simulink model "het_platoon_model"  (R2018b)
settings: Solver=ode1  StartTime=0.0  StopTime=simDrv.time_s(end)  FixedStep=sim_t_step  RelTol=1e-3
values from neighbouring files (symbols this model uses):
  sim_t_step = 0.01    [startHetPlatoonModel.m]
undefined symbols (not defined in the file or in its folder): adj_motEffMap, CTModel, DiscIntNeverNeededParam, LT, motSpdVec, motTrqVec, msk_mot_cont_trq, msk_mot_num, msk_mot_spd_bpt, MT, N_OptResults, simDrv, SPHETModel, TT
libraries: platooning_custom_blocks x24, simulink x7, dspstat3 x1, custom_func x1
(part 2 of 3)

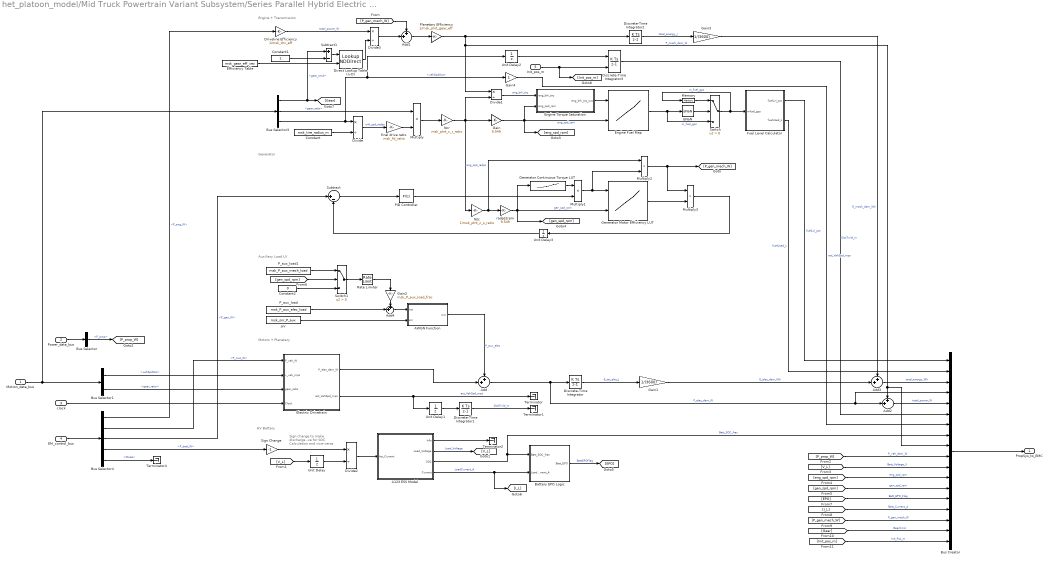
== system het_platoon_model/Mid Truck Powertrain Variant Subsystem/Series Parallel Hybrid Electric Truck/Series Parallel Hybrid Electric Powertrain Power Loss Model ==
  note: Sign change to make discharge -ve
      | for SOC Calculation and vice-versa
  note: Engine + Transmission
  note: HV Battery
  note: Auxiliary Load LV
  note: Motors + Planetary
  note: Generator
  Motion_data_bus : Inport
  Power_data_bus : Inport  Port=2
  clock : Inport  Port=3
  EM_control_bus : Inport  Port=4
  Init_pos_m : Inport  Port=5
  A123 ESS Model : Subsystem
  AWGN Function : MATLAB Function  TreatAsAtomicUnit=on
  Add{,1..4} (5 alike) : Sum  Inputs=++|
  Battery EPO Logic : Subsystem
  Bus Creator : BusCreator  Inputs=18
  Bus Selector : BusSelector  OutputSignals=P_prop
  Bus Selector1 : BusSelector  OutputSignals=vehSpdOut,gear_ratio
  Bus Selector3 : BusSelector  OutputSignals=gear_cmd,gear_ratio,vehSpdOut
  Bus Selector4 : BusSelector  OutputSignals=P_eng_W,P_mot_W,P_gen_W,P_batt_W,Mode
  Constant : Constant  Value=msk_tire_radius_m
  Constant1 : Constant
  Constant2 : Constant  Value=0
  Direct Lookup Table (n-D) : LookupNDDirect  NumberOfTableDimensions=1  TableIsInput=on
  Discrete-Time Integrator : DiscreteIntegrator  SampleTime=msk_t_step  ICPrevOutput=DiscIntNeverNeededParam  ICPrevScaledInput=DiscIntNeverNeededParam
  Discrete-Time Integrator1 : DiscreteIntegrator  SampleTime=msk_t_step  ICPrevOutput=DiscIntNeverNeededParam  ICPrevScaledInput=DiscIntNeverNeededParam
  Discrete-Time Integrator2 : DiscreteIntegrator  SampleTime=-1  ICPrevOutput=DiscIntNeverNeededParam  ICPrevScaledInput=DiscIntNeverNeededParam
  Discrete-Time Integrator3 : DiscreteIntegrator  InitialConditionSource=external  SampleTime=msk_t_step  ICPrevOutput=DiscIntNeverNeededParam  ICPrevScaledInput=DiscIntNeverNeededParam
  Divide{,1..3} (4 alike) : Product  Inputs=*/
  Driveline Efficiency : Gain  Gain=1/msk_drv_eff
  Efficiency Table : Constant  Value=msk_gear_eff_vec
  Electric Drivetrain : Subsystem
  Engine Fuel Map : Lookup_n-D  BreakpointsForDimension1=msk_eng_trq_bpt  BreakpointsForDimension2=msk_eng_spd_bpt  Table=msk_eng_fuel_map  ExtrapMethod=Clip  UseLastTableValue=on  InternalRulePriority=Speed  RndMeth=Simplest  InputSameDT=on
  Engine Torque Saturation : Subsystem
  Fuel Level Calculator : Subsystem
  Gain : Gain  Gain=9.549
  Gain1 : Gain  Gain=1/(3600)
  Gain2 : Gain  Gain=msk_P_aux_load_frac
  Gain3 : Gain  Gain=1/(3600)
  Gain4 : Gain
  Generator Continuous Torque LUT : Lookup_n-D  NumberOfTableDimensions=1  BreakpointsForDimension1=msk_gen_mtr_spdbpt  Table=msk_gen_mtr_cont_trq  InternalRulePriority=Speed  RndMeth=Simplest  InputSameDT=on
  Generator Motor Efficiency LUT : Lookup_n-D  BreakpointsForDimension1=msk_gen_mtr_trqbpt  BreakpointsForDimension2=msk_gen_mtr_spdbpt  Table=msk_gen_mtr_eff_map  ExtrapMethod=Clip  UseLastTableValue=on  InternalRulePriority=Speed  RndMeth=Simplest  InputSameDT=on
  IsNaN : RelationalOperator  Operator=isNaN  OutDataTypeStr=boolean  RndMeth=Simplest
  Memory : Memory
  Multiply{,1..3} (4 alike) : Product
  Ncr : Gain  Gain=msk_plnt_c_r_ratio
  Nsc : Gain  Gain=1/msk_plnt_c_s_ratio
  PID Controller : simulink/Continuous/PID Controller  Controller=PI  Form=Parallel  TimeDomain=Discrete-time  SampleTime=-1  IntegratorMethod=Forward Euler  FilterMethod=Forward Euler  ControllerParametersSource=internal  P=msk_gen_ctl_Kp  I=msk_gen_ctl_Ki  D=0  UseFilter=on  N=100  TunerSelectOption=Transfer Function Based (PID Tuner App)  InitialConditionSource=internal  InitialConditionForIntegrator=0  InitialConditionForFilter=0  DifferentiatorICPrevScaledInput=0  ExternalReset=none  TrackingMode=off  Kt=1  LimitOutput=on  UpperSaturationLimit=1  LowerSaturationLimit=0  LinearizeAsGain=on  AntiWindupMode=clamping  Kb=1  POutMin=[]  POutMax=[]  IOutMin=[]  IOutMax=[]  DOutMin=[]  DOutMax=[]  NOutMin=[]  NOutMax=[]  SumOutMin=[]  SumOutMax=[]  SaturationOutMin=[]  SaturationOutMax=[]  PParamMin=[]  PParamMax=[]  IParamMin=[]  IParamMax=[]  DParamMin=[]  DParamMax=[]  NParamMin=[]  NParamMax=[]  KbParamMin=[]  KbParamMax=[]  KtParamMin=[]  KtParamMax=[]  KbOutMin=[]  KbOutMax=[]  KtOutMin=[]  KtOutMax=[]  IntegratorOutMin=[]  IntegratorOutMax=[]  FilterOutMin=[]  FilterOutMax=[]  SumI1OutMin=[]  SumI1OutMax=[]  SumI2OutMin=[]  SumI2OutMax=[]  SumI3OutMin=[]  SumI3OutMax=[]  SumI4OutMin=[]  SumI4OutMax=[]  SumDOutMin=[]  SumDOutMax=[]  DifferentiatorOutMin=[]  DifferentiatorOutMax=[]  FilterDiffOutCoefMin=[]  FilterDiffOutCoefMax=[]  ReciprocalOutMin=[]  ReciprocalOutMax=[]  SumDenOutMin=[]  SumDenOutMax=[]  SumNumOutMin=[]  SumNumOutMax=[]  DivideOutMin=[]  DivideOutMax=[]  IntegratorContinuousStateAttributes=''  IntegratorStateMustResolveToSignalObject=off  IntegratorRTWStateStorageClass=Auto  FilterContinuousStateAttributes=''  FilterStateMustResolveToSignalObject=off  FilterRTWStateStorageClass=Auto  ParallelPVariant=InternalParameters  IdealPVariant=Disabled  IVariant=InternalParameters  DVariant=Disabled  IntegratorVariant=Discrete  SatVariant=Enabled  AWVariant=DiscClampingParallel  PCopyVariant=Disabled  TRVariant=Disabled  FdbkBlocksVariant=Forward  IdealPFdbkVariant=Disabled  SatFdbkVariant=Disabled  DerivativeFilterVariant=Disabled  NVariant=Disabled  NCopyVariant=Disabled_SignalSpec  FilterICVariant=Disabled  IntegratorICVariant=InternalICs  ExternalResetVariant=Disabled  TRSumVariant=Passthrough  SumFdbkVariant=Disabled  SumVariant=Sum_PI
  P_aux_load : Constant  Value=msk_P_aux_elec_load
  P_aux_load1 : Constant  Value=msk_P_aux_mech_load
  Planetary Efficiency : Gain  Gain=1/msk_plnt_gear_eff
  Rate Limiter : RateLimiter  RisingSlewLimit=100  FallingSlewLimit=-100  SampleTimeMode=inherited
  Sign Change : Gain  Gain=-1
  Subtract : Sum  Inputs=|+-
  Subtract1 : Sum  Inputs=+-
  Switch : Switch  Criteria=u2 > Threshold
  Switch1 : Switch  Criteria=u2 > Threshold
  Terminator{,1..2,4} (4 alike) : Terminator
  Unit Delay : UnitDelay  InitialCondition=msk_batt_Ns* msk_batt_Nmod * msk_cell_Vnom  SampleTime=-1
  Unit Delay1 : UnitDelay  SampleTime=-1
  Unit Delay2 : UnitDelay  SampleTime=-1
  Unit Delay3 : UnitDelay  SampleTime=-1
  final drive ratio : Gain  Gain=msk_fd_ratio
  radps2rpm : Gain  Gain=9.549
  snr : Constant  Value=msk_snr_P_aux
  PropSys_to_EMC : Outport
  wires:
  Divide3/1 -> Add1/2
  Bus Selector3/2 -> Multiply/1  "<gear_ratio>"
  Direct Lookup Table (n-D)/1 -> Divide3/2
  Efficiency Table/1 -> Direct Lookup Table (n-D)/2
  Constant1/1 -> Subtract1/2
  Subtract1/1 -> Direct Lookup Table (n-D)/1
  Add3/1 -> Bus Creator/3  "total_energy_Wh"
  Add2/1 -> Bus Creator/5  "total_power_W"
  Add1/1 -> Planetary Efficiency/1
  Bus Selector1/2 -> Electric Drivetrain/3(gear_ratio)  "<gear_ratio>"
  Driveline Efficiency/1 -> Divide3/1  "total_power_W"
  [P_gen_mech_W] -> Add1/1
  Unit Delay3/1 -> Subtract/2
  Multiply3/1 -> Unit Delay3/1
  Multiply2/1 -> Multiply3/1, [P_gen_mech_W]
  Generator Motor Efficiency LUT/1 -> Multiply3/2
  Generator Continuous Torque LUT/1 -> Multiply1/1
  Multiply1/1 -> Generator Motor Efficiency LUT/1, Multiply2/2
  PID Controller/1 -> Multiply1/2
  Subtract/1 -> PID Controller/1
  radps2rpm/1 -> [gen_spd_rpm], Generator Motor Efficiency LUT/2, Generator Continuous Torque LUT/1  "gen_spd_rpm"
  Nsc/1 -> radps2rpm/1, Multiply2/1
  Bus Selector4/2 -> Electric Drivetrain/1(P_veh_W)  "<P_mot_W>"
  Bus Selector/1 -> [P_prop_W]  "<P_prop>"
  EM_control_bus/1 -> Bus Selector4/1
  final drive ratio/1 -> Multiply/2
  Unit Delay2/1 -> Discrete-Time Integrator3/1
  Bus Selector3/3 -> Divide/1, Unit Delay2/1, Gain4/1  "<vehSpdOut>"
  Divide/1 -> final drive ratio/1  "whl_spd_radps"
  Gain4/1 -> Bus Creator/7  "act_VehSpd_mps"
  Discrete-Time Integrator3/1 -> Bus Creator/6  "DistTrvld_m"
  Divide1/1 -> Engine Torque Saturation/1(eng_brk_trq)  "eng_brk_trq"
  Fuel Level Calculator/2(fuelUsed_L) -> Bus Creator/2  "fuelUsed_L"
  Multiply/1 -> Ncr/1
  Discrete-Time Integrator2/1 -> Gain3/1  "total_energy_J"
  Engine Torque Saturation/1(eng_brk_trq_out) -> Engine Fuel Map/1
  Fuel Level Calculator/1(fuelLvl_pct) -> Bus Creator/1  "fuelLvl_pct"
  Motion_data_bus/1 -> Bus Selector1/1, Bus Selector3/1
  Gain3/1 -> Add3/1  "E_mech_dem_Wh"
  Constant/1 -> Divide/2
  Gain/1 -> [eng_spd_rpm], Engine Fuel Map/2, Engine Torque Saturation/2(eng_spd_rpm)  "eng_spd_rpm"
  Unit Delay1/1 -> Discrete-Time Integrator1/1
  Discrete-Time Integrator1/1 -> Terminator1/1  "DistTrvld_m"
  Electric Drivetrain/2(act_VehSpd_mps) -> Unit Delay1/1, Terminator/1  "act_VehSpd_mps"
  A123 ESS Model/4(Current) -> [I_L], Battery EPO Logic/2(LoadCurrent_A)  "LoadCurrent_A"
  Bus Selector4/4 -> Sign Change/1  "<P_batt_W>"
  Sign Change/1 -> Divide2/1
  Battery EPO Logic/1(Batt_EPO) -> [EPO]  "BattEPOFlag"
  Unit Delay/1 -> Divide2/2
  [V_L] -> Unit Delay/1
  A123 ESS Model/1(Info) -> Terminator2/1
  A123 ESS Model/3(SOC) -> Battery EPO Logic/1(Batt_SOC_frac), Bus Creator/8  "Batt_SOC_frac"
  Divide2/1 -> A123 ESS Model/1(Inp_Current)
  A123 ESS Model/2(Load_Voltage) -> [V_L]  "Load_Voltage"
  Gain1/1 -> Add3/2  "E_elec_dem_Wh"
  Discrete-Time Integrator/1 -> Gain1/1  "E_tot_elec_J"
  Bus Creator/1 -> PropSys_to_EMC/1
  Electric Drivetrain/1(P_elec_dem_W) -> Add/2
  Add/1 -> Bus Creator/4, Add2/2, Discrete-Time Integrator/1  "P_elec_dem_W"
  AWGN Function/1(out) -> Add/1  "P_aux_elec"
  snr/1 -> AWGN Function/2(snr)
  P_aux_load/1 -> Add4/2
  Bus Selector1/1 -> Electric Drivetrain/2(v_veh_mps)  "<vehSpdOut>"
  clock/1 -> Electric Drivetrain/4(Clock)
  Power_data_bus/1 -> Bus Selector/1
  Bus Selector3/1 -> Subtract1/1, [Gear]  "<gear_cmd>"
  Switch/1 -> Fuel Level Calculator/1(mfuel_gps), Memory/1  "m_fuel_gps"
  Memory/1 -> Switch/1
  Engine Fuel Map/1 -> Switch/3, IsNaN/1  "m_fuel_gps"
  IsNaN/1 -> Switch/2
  [P_prop_W] -> Bus Creator/10  "P_veh_dem_W"
  Bus Selector4/1 -> Driveline Efficiency/1  "<P_eng_W>"
  Bus Selector4/3 -> Subtract/1  "<P_gen_W>"
  Bus Selector4/5 -> Terminator4/1  "<Mode>"
  [V_L] -> Bus Creator/11  "Batt_Voltage_V"
  Ncr/1 -> Divide1/2, Gain/1, Nsc/1  "eng_spd_radps"
  [gen_spd_rpm] -> Bus Creator/13  "gen_spd_rpm"
  [eng_spd_rpm] -> Bus Creator/12  "eng_spd_rpm"
  Init_pos_m/1 -> [Init_pos_m], Discrete-Time Integrator3/2
  Add4/1 -> AWGN Function/1(inp)
  Gain2/1 -> Add4/1
  P_aux_load1/1 -> Switch1/1
  Switch1/1 -> Rate Limiter/1
  Rate Limiter/1 -> Gain2/1
  [gen_spd_rpm] -> Switch1/2
  Constant2/1 -> Switch1/3
  [Gear] -> Bus Creator/17  "GearCmd"
  [EPO] -> Bus Creator/14  "Batt_EPO_Flag"
  [I_L] -> Bus Creator/15  "Batt_Current_A"
  [P_gen_mech_W] -> Bus Creator/16  "P_gen_mech_W"
  Planetary Efficiency/1 -> Divide1/1, Bus Creator/9, Add2/1, Discrete-Time Integrator2/1  "P_mech_dem_W"
  [Init_pos_m] -> Bus Creator/18  "Init_Pos_m"

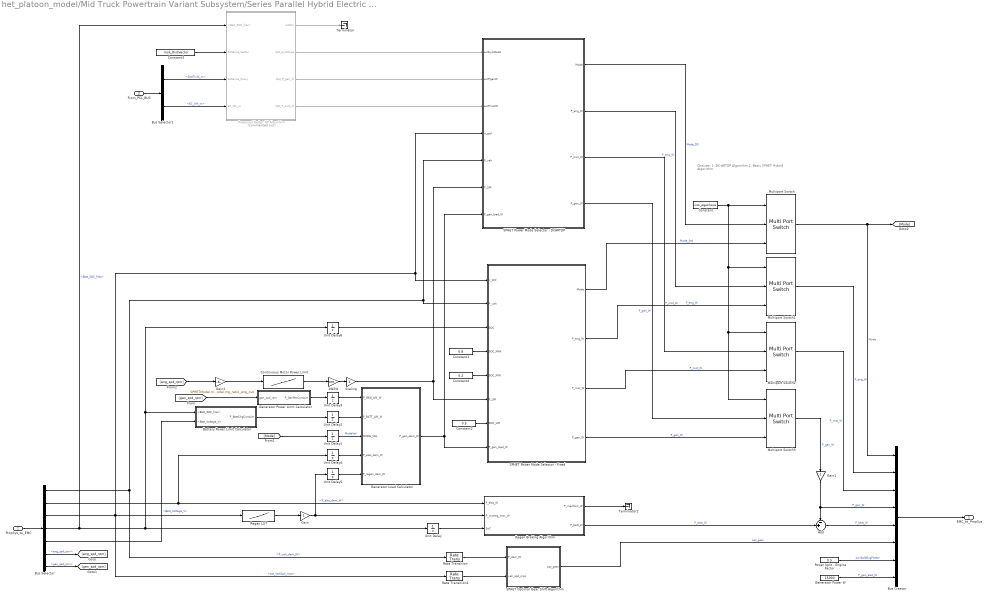
== system het_platoon_model/Mid Truck Powertrain Variant Subsystem/Series Parallel Hybrid Electric Truck/Series Parallel Hybrid Electric Truck Energy Management System ==
  note: Choices:
      | 1: DC-ARTDP Algorithm
      | 2: Basic SPHET Hybrid Algorithm
  PropSys_to_EMC : Inport
  From_PCL_BUS : Inport  Port=2
  Add : Sum  Inputs=-+|
  Battery Power Limit Calculator : Subsystem
  Bus Creator : BusCreator  Inputs=8
  Bus Selector : BusSelector  OutputSignals=P_veh_dem_W,P_elec_dem_W,act_VehSpd_mps,Batt_SOC_frac,Batt_Voltage_V,eng_spd_rpm,gen_spd_rpm
  Bus Selector1 : BusSelector  OutputSignals=DistTrvld_m,EC_Wh_m
  Constant : Constant  Value=msk_algoChoice
  Constant1 : Constant  Value=0.8
  Constant2 : Constant  Value=0.5
  Constant3 : Constant  Value=msk_DistVector
  Constant4 : Constant  Value=0.2
  Continuous Motor Power Limit : Lookup_n-D  NumberOfTableDimensions=1  BreakpointsForDimension1=SPHETModel.cont_mtr_trq_spdbpt  Table=SPHETModel.cont_mtr_pwr_map  InternalRulePriority=Speed  RndMeth=Simplest  InputSameDT=on
  Gain : Gain  Gain=-1
  Gain1 : Gain
  Gain2 : Gain  Gain=SPHETModel.mg_ratio_mot_out/SPHETModel.mg_ratio_eng_out
  Generator Load Calculator : MATLAB Function  TreatAsAtomicUnit=on
  Generator Power Limit Calculator : Subsystem
  Generator Power W : Constant  Value=15000
  Multiport Switch{,1..3} (4 alike) : MultiPortSwitch  Inputs=2
  Power Split - Engine Factor : Constant  Value=0.5
  Proposed ReOpt DP Algorithm : Subsystem  Commented=on
  Rate Transition : RateTransition  OutPortSampleTime=sim_t_step
  Rate Transition1 : RateTransition  OutPortSampleTime=sim_t_step
  Regen Braking Algorithm : Stateflow chart  TreatAsAtomicUnit=on
  Regen LUT : Lookup_n-D  NumberOfTableDimensions=1  BreakpointsForDimension1=msk_regen_spd_bpt  Table=msk_regen_pwr_vec*-1  ExtrapMethod=Clip  UseLastTableValue=on  InternalRulePriority=Speed  RndMeth=Simplest  InputSameDT=on
  SPHET Optimal Gear Shift Algorithm : Subsystem  mask{msk_tire_radius_m=SPHETModel.ld_tire_rad_m, msk_trns_eff_avg=mean(SPHETModel.gear_eff) * SPHETModel.plnt_gear_eff, msk_init_gear=1}
      mask prompts: msk_tire_radius_m "Vehicle tire radius :"; msk_trns_eff_avg "Average transmission efficiency :"; msk_init_gear "Initial gear selection :"
      mask DialogControl DescGroupVar Prompt: Optimal Gear Shift Algorithm
      mask DialogControl DescTextVar Prompt: The block computes optimal gear based on the power demand and vehicle speed by minimizing fuel consumption.
  SPHET Power Mode Selector - DCARTDP : Stateflow chart  TreatAsAtomicUnit=on
  SPHET Power Mode Selector - Fixed : Stateflow chart  TreatAsAtomicUnit=on
  Scaling : Gain
  Terminator : Terminator
  Terminator2 : Terminator
  Unit Delay{,1..6} (7 alike) : UnitDelay  SampleTime=-1
  kW2W : Gain  Gain=1000
  EMC_to_PropSys : Outport
  wires:
  Bus Selector/1 -> SPHET Power Mode Selector - DCARTDP/5(P_veh), SPHET Power Mode Selector - Fixed/2(P_veh), Rate Transition/1  "<P_veh_dem_W>"
  Generator Power W/1 -> Bus Creator/8  "P_gen_elec_W"
  Power Split - Engine Factor/1 -> Bus Creator/7  "pwrSplitEngFactor"
  Bus Creator/1 -> EMC_to_PropSys/1
  From_PCL_BUS/1 -> Bus Selector1/1
  PropSys_to_EMC/1 -> Bus Selector/1
  Bus Selector/4 -> Proposed ReOpt DP Algorithm/1(<Batt_SOC_frac>), Battery Power Limit Calculator/1(<Batt_SOC_frac>), Unit Delay6/1, Unit Delay/1  "<Batt_SOC_frac>"
  Bus Selector/2 -> Regen Braking Algorithm/1(P_elec_W), Unit Delay4/1  "<P_elec_dem_W>"
  Add/1 -> Bus Creator/5  "P_batt_W"
  Regen LUT/1 -> Gain/1
  Regen Braking Algorithm/1(P_mechbrk_W) -> Terminator2/1
  Unit Delay/1 -> Regen Braking Algorithm/3(SoC)
  Bus Selector/3 -> Regen LUT/1, SPHET Power Mode Selector - DCARTDP/4(v_spd), SPHET Power Mode Selector - Fixed/1(v_spd), Rate Transition1/1  "<act_VehSpd_mps>"
  Rate Transition/1 -> SPHET Optimal Gear Shift Algorithm/1(P_dem_W)
  Rate Transition1/1 -> SPHET Optimal Gear Shift Algorithm/2(veh_spd_mps)
  SPHET Optimal Gear Shift Algorithm/1(opt_gear) -> Bus Creator/6  "opt_gear"
  kW2W/1 -> Scaling/1
  Constant1/1 -> SPHET Power Mode Selector - Fixed/4(SOC_MAX)
  Constant2/1 -> SPHET Power Mode Selector - Fixed/7(SOC_LIM)
  Multiport Switch/1 -> Bus Creator/1, [Mode]  "Mode"
  Regen Braking Algorithm/2(P_batt_W) -> Add/2  "P_batt_W"
  Multiport Switch3/1 -> Gain1/1  "P_gen_W"
  Multiport Switch1/1 -> Bus Creator/2  "P_eng_W"
  Multiport Switch2/1 -> Bus Creator/3  "P_mot_W"
  Generator Load Calculator/1(P_gen_dem_W) -> SPHET Power Mode Selector - DCARTDP/7(P_gen_load_W), SPHET Power Mode Selector - Fixed/8(P_gen_load_W)
  Bus Selector/6 -> [eng_spd_rpm]  "<eng_spd_rpm>"
  Bus Selector/7 -> [gen_spd_rpm]  "<gen_spd_rpm>"
  [Mode] -> Unit Delay1/1
  Unit Delay1/1 -> Generator Load Calculator/3(MODE_VAL)  "ModeVal"
  Bus Selector/5 -> Battery Power Limit Calculator/2(<Batt_Voltage_V>)  "<Batt_Voltage_V>"
  Battery Power Limit Calculator/1(P_BattChgContLim) -> Unit Delay2/1
  [gen_spd_rpm] -> Generator Power Limit Calculator/1(gen_spd_rpm)
  Generator Power Limit Calculator/1(P_GenMtrContLim) -> Unit Delay3/1
  Gain/1 -> Regen Braking Algorithm/2(P_motreg_max_W), Unit Delay5/1
  Gain1/1 -> Add/1, Bus Creator/4  "P_gen_W"
  Unit Delay2/1 -> Generator Load Calculator/2(P_BATT_LIM_W)
  Unit Delay3/1 -> Generator Load Calculator/1(P_GEN_LIM_W)
  Unit Delay4/1 -> Generator Load Calculator/4(P_elec_dem_W)
  Unit Delay5/1 -> Generator Load Calculator/5(P_regen_dem_W)
  Unit Delay6/1 -> SPHET Power Mode Selector - Fixed/3(SOC)
  Continuous Motor Power Limit/1 -> kW2W/1
  Gain2/1 -> Continuous Motor Power Limit/1
  [eng_spd_rpm] -> Gain2/1
  SPHET Power Mode Selector - Fixed/4(P_gen_W) -> Multiport Switch3/3  "P_gen_W"
  SPHET Power Mode Selector - Fixed/3(P_mot_W) -> Multiport Switch2/3  "P_mot_W"
  SPHET Power Mode Selector - Fixed/2(P_eng_W) -> Multiport Switch1/3  "P_eng_W"
  SPHET Power Mode Selector - Fixed/1(Mode) -> Multiport Switch/3  "Mode_Std"
  SPHET Power Mode Selector - DCARTDP/4(P_gen_W) -> Multiport Switch3/2  "P_gen_W"
  SPHET Power Mode Selector - DCARTDP/3(P_mot_W) -> Multiport Switch2/2  "P_mot_W"
  SPHET Power Mode Selector - DCARTDP/2(P_eng_W) -> Multiport Switch1/2  "P_eng_W"
  SPHET Power Mode Selector - DCARTDP/1(Mode) -> Multiport Switch/2  "Mode_DC"
  Constant/1 -> Multiport Switch3/1, Multiport Switch2/1, Multiport Switch1/1, Multiport Switch/1
  Bus Selector1/2 -> Proposed ReOpt DP Algorithm/4(EC_Wh_m)  "<EC_Wh_m>"
  Bus Selector1/1 -> Proposed ReOpt DP Algorithm/3(Distance_Query)  "<DistTrvld_m>"
  Proposed ReOpt DP Algorithm/4(Opt_P_mot_W) -> SPHET Power Mode Selector - DCARTDP/3(extPmotW)
  Proposed ReOpt DP Algorithm/2(Opt_HybMode) -> SPHET Power Mode Selector - DCARTDP/1(extHybMode)
  Proposed ReOpt DP Algorithm/3(Opt_P_gen_W) -> SPHET Power Mode Selector - DCARTDP/2(extPgenW)
  Proposed ReOpt DP Algorithm/1(distIdx) -> Terminator/1
  Constant3/1 -> Proposed ReOpt DP Algorithm/2(Distance_Vector)
  Scaling/1 -> SPHET Power Mode Selector - DCARTDP/6(P_LIM), SPHET Power Mode Selector - Fixed/6(P_LIM)
  Constant4/1 -> SPHET Power Mode Selector - Fixed/5(SOC_MIN)

== system het_platoon_model/Mid Truck Powertrain Variant Subsystem/Series Parallel Hybrid Electric Truck/Series Parallel Hybrid Electric Post-Processing/Blending Function 1 ==
  runAvgFuelEC_Wh_m : Inport
  Fuel_Used_L : Inport  Port=2
  stAvgFuelEC_Wh_m : Inport  Port=3
  Constant1 : Constant  Value=msk_fuel_init_liters
  Divide : Product  Inputs=*/
  Product1 : Product
  Subtract1 : Sum  Inputs=-+
  Subtract2 : Sum
  blndElecEC_Wh_m : Outport
  wires:
  Subtract2/1 -> blndElecEC_Wh_m/1  "blndElecEC_Wh_m"
  Subtract1/1 -> Product1/2
  Product1/1 -> Subtract2/2
  Constant1/1 -> Divide/2
  Fuel_Used_L/1 -> Divide/1
  Divide/1 -> Product1/1
  stAvgFuelEC_Wh_m/1 -> Subtract1/2
  runAvgFuelEC_Wh_m/1 -> Subtract2/1, Subtract1/1

== system het_platoon_model/Mid Truck Powertrain Variant Subsystem/Series Parallel Hybrid Electric Truck/Series Parallel Hybrid Electric Post-Processing/Blending Function 2 ==
  runAvgFC_L_100km : Inport
  Fuel_Used_L : Inport  Port=2
  stAvgFC_L_100km : Inport  Port=3
  Constant1 : Constant  Value=msk_fuel_init_liters
  Divide : Product  Inputs=*/
  Product1 : Product
  Subtract1 : Sum  Inputs=-+
  Subtract2 : Sum
  blndFC_L_100km : Outport
  wires:
  Subtract2/1 -> blndFC_L_100km/1  "blndFC_L_100km"
  Divide/1 -> Product1/1
  Fuel_Used_L/1 -> Divide/1
  Constant1/1 -> Divide/2
  runAvgFC_L_100km/1 -> Subtract2/1, Subtract1/1
  stAvgFC_L_100km/1 -> Subtract1/2
  Product1/1 -> Subtract2/2
  Subtract1/1 -> Product1/2

== system het_platoon_model/Mid Truck Powertrain Variant Subsystem/Series Parallel Hybrid Electric Truck/Series Parallel Hybrid Electric Post-Processing/Distance to Empty Calculator ==
  note: Assuming 10% of the fuel in the tank
      | is not available for consumption.
  blndEC_Wh_m : Inport
  <fuelUsed_L> : Inport  Port=2
  battSOC_frac : Inport  Port=3
  Battery Energy Max : Constant  Value=msk_batt_Ns * msk_batt_Np * msk_batt_Nmod * msk_cell_Vnom * msk_cell_Q_Ah
  Constant : Constant  Value=msk_fuel_init_liters
  Constant1 : Constant  Value=0.2
  Divide : Product  Inputs=*/
  Fuel LHV energy per volume : Constant  Value=msk_fuel_rho_kgpl * msk_fuel_lhv_kwhpkg
  Percent of Fuel in Tank : Gain  Gain=0.9
  Product2 : Product
  Product3 : Product
  Subtract : Sum  Inputs=-+
  Subtract1 : Sum  Inputs=+-
  Subtract2 : Sum  Inputs=++|
  kWh2Wh : Gain  Gain=1000
  m2km : Gain  Gain=0.001
  estDTE_km : Outport
  wires:
  m2km/1 -> estDTE_km/1  "estDTE_km"
  Constant/1 -> Percent of Fuel in Tank/1
  Subtract/1 -> Product2/2
  <fuelUsed_L>/1 -> Subtract/1
  blndEC_Wh_m/1 -> Divide/2
  Percent of Fuel in Tank/1 -> Subtract/2
  Constant1/1 -> Subtract1/2
  battSOC_frac/1 -> Subtract1/1
  Fuel LHV energy per volume/1 -> Product2/1
  Product2/1 -> kWh2Wh/1
  Battery Energy Max/1 -> Product3/2
  Subtract1/1 -> Product3/1
  Product3/1 -> Subtract2/1
  kWh2Wh/1 -> Subtract2/2
  Subtract2/1 -> Divide/1
  Divide/1 -> m2km/1

== system het_platoon_model/Mid Truck Powertrain Variant Subsystem/Series Parallel Hybrid Electric Truck/Series Parallel Hybrid Electric Post-Processing/Fuel Consumption Calculator ==
  <fuelUsed_L> : Inport
  <DistTrvld_m> : Inport  Port=2
  Constant : Constant  Value=100
  Constant1 : Constant  Value=eps
  Divide1 : Product  Inputs=*/
  Divide2 : Product  Inputs=*/
  Switch : Switch  Criteria=u2 > Threshold
  m2km : Gain  Gain=1/1000
  FC_Lp100km : Outport
  wires:
  Constant/1 -> Divide2/1
  Constant1/1 -> Switch/3
  <fuelUsed_L>/1 -> Divide1/2
  m2km/1 -> Switch/2, Switch/1
  Divide1/1 -> Divide2/2
  Switch/1 -> Divide1/1
  <DistTrvld_m>/1 -> m2km/1
  Divide2/1 -> FC_Lp100km/1  "FC_Lp100km"

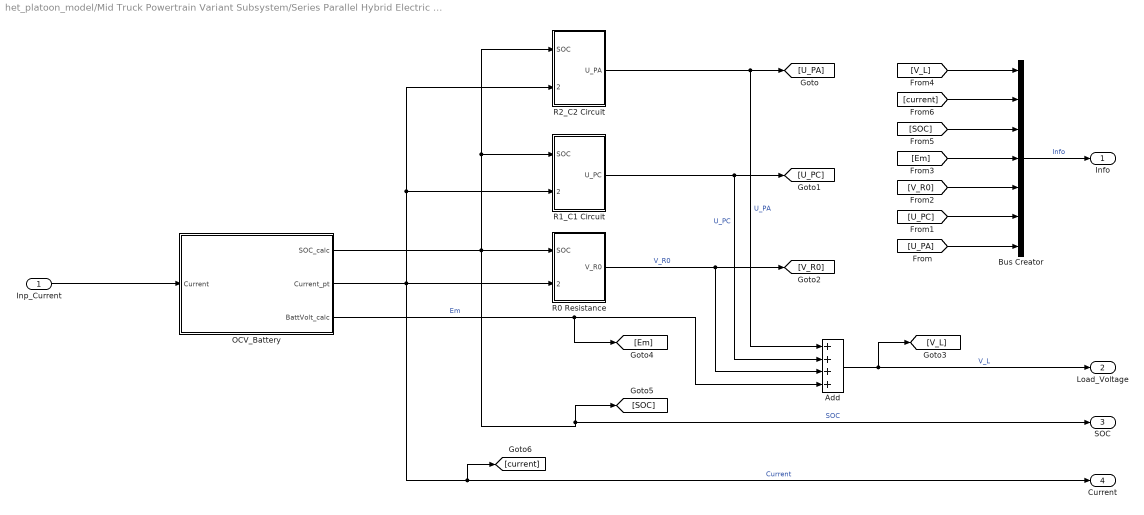
== system het_platoon_model/Mid Truck Powertrain Variant Subsystem/Series Parallel Hybrid Electric Truck/Series Parallel Hybrid Electric Powertrain Power Loss Model/A123 ESS Model ==
  Inp_Current : Inport
  Add : Sum  Inputs=++++
  Bus Creator : BusCreator  Inputs=7
  OCV_Battery : Subsystem
  R0 Resistance : Subsystem
  R1_C1 Circuit : Subsystem
  R2_C2 Circuit : Subsystem
  Info : Outport
  Load_Voltage : Outport  Port=2
  SOC : Outport  Port=3
  Current : Outport  Port=4
  wires:
  [V_L] -> Bus Creator/1
  Bus Creator/1 -> Info/1  "Info"
  [V_R0] -> Bus Creator/5
  OCV_Battery/3(BattVolt_calc) -> Add/4, [Em]  "Em"
  [U_PC] -> Bus Creator/6
  R1_C1 Circuit/1(U_PC) -> [U_PC], Add/2  "U_PC"
  OCV_Battery/1(SOC_calc) -> R0 Resistance/1(SOC), R1_C1 Circuit/1(SOC), R2_C2 Circuit/1(SOC), [SOC], SOC/1  "SOC"
  OCV_Battery/2(Current_pt) -> R0 Resistance/2(Current), R1_C1 Circuit/2(Current), R2_C2 Circuit/2(Current), [current], Current/1  "Current"
  R2_C2 Circuit/1(U_PA) -> [U_PA], Add/1  "U_PA"
  R0 Resistance/1(V_R0) -> Add/3, [V_R0]  "V_R0"
  [Em] -> Bus Creator/4
  Add/1 -> [V_L], Load_Voltage/1  "V_L"
  [current] -> Bus Creator/2
  Inp_Current/1 -> OCV_Battery/1(Current)
  [U_PA] -> Bus Creator/7
  [SOC] -> Bus Creator/3

== system het_platoon_model/Mid Truck Powertrain Variant Subsystem/Series Parallel Hybrid Electric Truck/Series Parallel Hybrid Electric Powertrain Power Loss Model/Battery EPO Logic ==
  note: Discharge Current is negative
  Batt_SOC_frac : Inport
  LoadCurrent_A : Inport  Port=2
  10-second average : dspstat3/Moving Average  Method=Sliding window  ForgettingFactorPort=off  SpecifyWindowLength=on  WindowLength=1000  ForgettingFactor=0.9  SimulateUsing=Code generation
  10sec Discharge Limit Table A123 : Lookup_n-D  BreakpointsForDimension1=msk_cellTempbpt  BreakpointsForDimension2=msk_soc_bpt  Table=msk_dchglim10s  ExtrapMethod=Clip  UseLastTableValue=on  InternalRulePriority=Speed  RndMeth=Simplest  InputSameDT=on
  Battery EPO Constraint Logic : Stateflow chart  TreatAsAtomicUnit=on
  CellTemp degC : Constant  Value=35
  Gain1 : Gain  Gain=-1
  Batt_EPO : Outport
  wires:
  10sec Discharge Limit Table A123/1 -> Gain1/1
  Gain1/1 -> Battery EPO Constraint Logic/1(DchgCurrLim)
  CellTemp degC/1 -> 10sec Discharge Limit Table A123/1
  10-second average/1 -> Battery EPO Constraint Logic/2(LoadCurr)  "LoadCurrent_10sAvg_A"
  Battery EPO Constraint Logic/1(epo_flag) -> Batt_EPO/1  "Batt_EPO"
  LoadCurrent_A/1 -> 10-second average/1
  Batt_SOC_frac/1 -> 10sec Discharge Limit Table A123/2

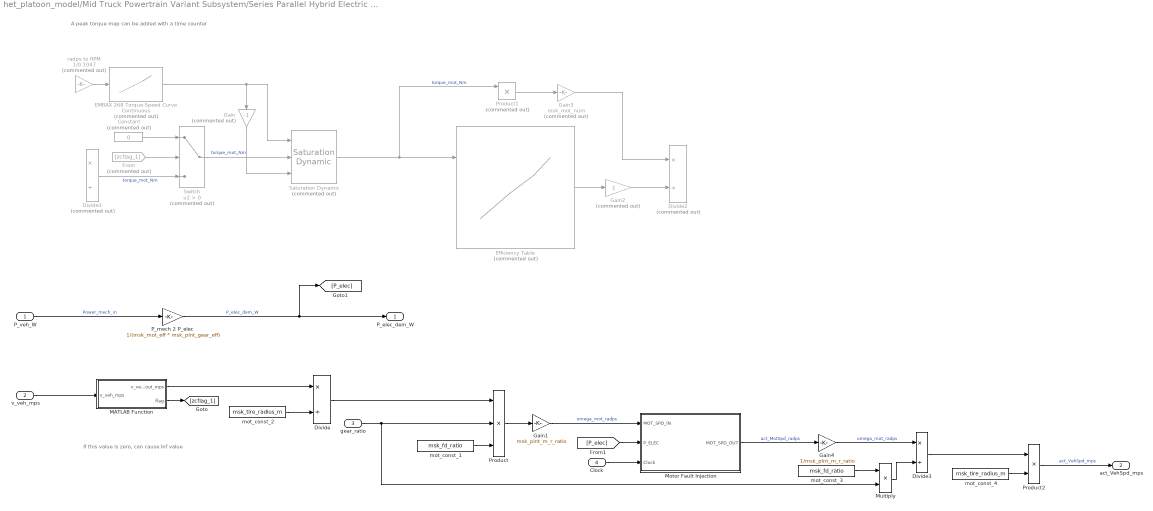
== system het_platoon_model/Mid Truck Powertrain Variant Subsystem/Series Parallel Hybrid Electric Truck/Series Parallel Hybrid Electric Powertrain Power Loss Model/Electric Drivetrain ==
  note: If this value is zero, can cause Inf value
  note: A peak torque map can be added with a time counter
  P_veh_W : Inport
  v_veh_mps : Inport  Port=2
  gear_ratio : Inport  Port=3
  Clock : Inport  Port=4
  Constant : Constant  Commented=on  Value=0
  Divide : Product  Inputs=*/
  Divide1 : Product  Commented=on  Inputs=*/
  Divide2 : Product  Commented=on  Inputs=*/
  Divide3 : Product  Inputs=*/
  EMRAX 268 Torque-Speed Curve Continuous : Lookup_n-D  Commented=on  NumberOfTableDimensions=1  BreakpointsForDimension1=msk_mot_spd_bpt  Table=msk_mot_cont_trq  InternalRulePriority=Speed  RndMeth=Simplest  InputSameDT=on
  Efficiency Table : Lookup_n-D  Commented=on  BreakpointsForDimension1=motTrqVec  BreakpointsForDimension2=motSpdVec  Table=adj_motEffMap  ExtrapMethod=Clip  UseLastTableValue=on  InternalRulePriority=Speed  RndMeth=Simplest  InputSameDT=on
  From : From  Commented=on  GotoTag=zcflag_1
  Gain : Gain  Commented=on  Gain=-1
  Gain1 : Gain  Gain=msk_plnt_m_r_ratio
  Gain2 : Gain  Commented=on
  Gain3 : Gain  Commented=on  Gain=msk_mot_num
  Gain4 : Gain  Gain=1/msk_plnt_m_r_ratio
  MATLAB Function : MATLAB Function  TreatAsAtomicUnit=on
  Motor Fault Injection : Subsystem  mask{FaultDec=off, P_derate=30000, t_fault=6000, contMotTrqMax=180}
      mask prompts: FaultDec "Select to enable motor deration fault."; P_derate "Enter the motor deration power [Watts]:"; t_fault "Time for fault insertion [seconds]:"; contMotTrqMax "Maximum Continuous Motor Torque [Nm]:"
      mask DialogControl DescGroupVar Prompt: Motor Fault Injection
      mask DialogControl DescTextVar Prompt: Use the parameter controls to induce a deration fault in the motor subsystem.
  Multiply : Product
  P_mech 2 P_elec : Gain  Gain=1/(msk_mot_eff * msk_plnt_gear_eff)
  Product : Product  Inputs=3
  Product1 : Product  Commented=on
  Product2 : Product
  Saturation Dynamic : simulink/Discontinuities/Saturation Dynamic  Commented=on  OutMin=[]  OutMax=[]  OutDataTypeStr=Inherit: Same as second input  OutDataType=fixdt(1, 16)  OutScaling=2^-10  DoSatur=off
  Switch : Switch  Commented=on  Criteria=u2 > Threshold
  mot_const_1 : Constant  Value=msk_fd_ratio
  mot_const_2 : Constant  Value=msk_tire_radius_m
  mot_const_3 : Constant  Value=msk_fd_ratio
  mot_const_4 : Constant  Value=msk_tire_radius_m
  radps to RPM : Gain  Commented=on  Gain=1/0.1047
  P_elec_dem_W : Outport
  act_VehSpd_mps : Outport  Port=2
  wires:
  Multiply/1 -> Divide3/2
  Gain4/1 -> Divide3/1  "omega_mot_radps"
  Product/1 -> Gain1/1
  mot_const_1/1 -> Product/3
  Divide/1 -> Product/1
  Product2/1 -> act_VehSpd_mps/1  "act_VehSpd_mps"
  mot_const_4/1 -> Product2/2
  Divide3/1 -> Product2/1
  mot_const_3/1 -> Multiply/1
  Clock/1 -> Motor Fault Injection/3(Clock)
  [P_elec] -> Motor Fault Injection/2(P_ELEC)
  Gain1/1 -> Motor Fault Injection/1(MOT_SPD_IN)  "omega_mot_radps"
  Motor Fault Injection/1(MOT_SPD_OUT) -> Gain4/1  "act_MotSpd_radps"
  Divide1/1 -> Switch/3  "torque_mot_Nm"
  Gain3/1 -> Divide2/1
  Gain2/1 -> Divide2/2
  P_mech 2 P_elec/1 -> P_elec_dem_W/1, [P_elec]  "P_elec_dem_W"
  Product1/1 -> Gain3/1
  MATLAB Function/2(flag) -> [zcflag_1]
  mot_const_2/1 -> Divide/2
  Switch/1 -> Saturation Dynamic/2  "torque_mot_Nm"
  Efficiency Table/1 -> Gain2/1
  v_veh_mps/1 -> MATLAB Function/1(v_veh_mps)
  P_veh_W/1 -> P_mech 2 P_elec/1  "Power_mech_in"
  EMRAX 268 Torque-Speed Curve Continuous/1 -> Saturation Dynamic/1, Gain/1
  gear_ratio/1 -> Product/2, Multiply/2
  Gain/1 -> Saturation Dynamic/3
  Constant/1 -> Switch/1
  radps to RPM/1 -> EMRAX 268 Torque-Speed Curve Continuous/1
  MATLAB Function/1(v_veh_out_mps) -> Divide/1
  From/1 -> Switch/2
  Saturation Dynamic/1 -> Efficiency Table/1, Product1/1  "torque_mot_Nm"

== system het_platoon_model/Mid Truck Powertrain Variant Subsystem/Series Parallel Hybrid Electric Truck/Series Parallel Hybrid Electric Powertrain Power Loss Model/Engine Torque Saturation ==
  eng_brk_trq : Inport
  eng_spd_rpm : Inport  Port=2
  Engine Peak Motoring Torque LUT : Lookup_n-D  NumberOfTableDimensions=1  BreakpointsForDimension1=msk_eng_trq_spd_bpt  Table=msk_eng_pk_mtr_trq  ExtrapMethod=Clip  UseLastTableValue=on  InternalRulePriority=Speed  RndMeth=Simplest  InputSameDT=on
  "Engine Peak Propulsion Torque LUT " : Lookup_n-D  NumberOfTableDimensions=1  BreakpointsForDimension1=msk_eng_trq_spd_bpt  Table=msk_eng_pk_trq_vec  ExtrapMethod=Clip  UseLastTableValue=on  InternalRulePriority=Speed  RndMeth=Simplest  InputSameDT=on
  Saturation Dynamic : simulink/Discontinuities/Saturation Dynamic  OutMin=[]  OutMax=[]  OutDataTypeStr=Inherit: Same as second input  OutDataType=fixdt(1, 16)  OutScaling=2^-10  DoSatur=off
  eng_brk_trq_out : Outport
  wires:
  "Engine Peak Propulsion Torque LUT "/1 -> Saturation Dynamic/1
  Engine Peak Motoring Torque LUT/1 -> Saturation Dynamic/3
  eng_spd_rpm/1 -> Engine Peak Motoring Torque LUT/1, "Engine Peak Propulsion Torque LUT "/1
  Saturation Dynamic/1 -> eng_brk_trq_out/1
  eng_brk_trq/1 -> Saturation Dynamic/2

== system het_platoon_model/Mid Truck Powertrain Variant Subsystem/Series Parallel Hybrid Electric Truck/Series Parallel Hybrid Electric Powertrain Power Loss Model/Fuel Level Calculator ==
  mfuel_gps : Inport
  Constant : Constant  Value=msk_fuel_init_liters
  Discrete-Time Integrator : DiscreteIntegrator  SampleTime=msk_t_step  ICPrevOutput=DiscIntNeverNeededParam  ICPrevScaledInput=DiscIntNeverNeededParam
  Divide1 : Product  Inputs=*/
  Fuel Density : Gain  Gain=(0.001/msk_rho_fuel_kgpL)
  Gain1 : Gain  Gain=100
  Subtract : Sum  Inputs=+-
  fuelLvl_pct : Outport
  fuelUsed_L : Outport  Port=2
  wires:
  Gain1/1 -> fuelLvl_pct/1  "fuelLvl_pct"
  mfuel_gps/1 -> Discrete-Time Integrator/1
  Discrete-Time Integrator/1 -> Fuel Density/1  "mfuel_g"
  Constant/1 -> Subtract/1, Divide1/2
  Fuel Density/1 -> Subtract/2, fuelUsed_L/1  "fuelUsed_liters"
  Subtract/1 -> Divide1/1  "fuelLeft_liters"
  Divide1/1 -> Gain1/1

== system het_platoon_model/Mid Truck Powertrain Variant Subsystem/Series Parallel Hybrid Electric Truck/Series Parallel Hybrid Electric Truck Energy Management System/Battery Power Limit Calculator ==
  <Batt_SOC_frac> : Inport
  <Batt_Voltage_V> : Inport  Port=2
  Battery Continuous Charge Limit : Lookup_n-D  BreakpointsForDimension1=SPHETModel.cellTempbpt_C  BreakpointsForDimension2=SPHETModel.socbpt  Table=SPHETModel.ChgCurrLim_cont_A  ExtrapMethod=Clip  UseLastTableValue=on  InternalRulePriority=Speed  RndMeth=Simplest  InputSameDT=on
  Constant3 : Constant  Value=25
  Gain1 : Gain
  Multiply : Product
  P_BattChgContLim : Outport
  wires:
  <Batt_Voltage_V>/1 -> Multiply/2
  Constant3/1 -> Battery Continuous Charge Limit/1
  Gain1/1 -> Multiply/1
  Battery Continuous Charge Limit/1 -> Gain1/1
  <Batt_SOC_frac>/1 -> Battery Continuous Charge Limit/2
  Multiply/1 -> P_BattChgContLim/1  "P_BattChgContLim"

== system het_platoon_model/Mid Truck Powertrain Variant Subsystem/Series Parallel Hybrid Electric Truck/Series Parallel Hybrid Electric Truck Energy Management System/Generator Power Limit Calculator ==
  gen_spd_rpm : Inport
  Constant : Constant  Value=5000
  Divide : Product  Inputs=*/
  Gain : Gain
  Generator Continuous Power kW : Lookup_n-D  NumberOfTableDimensions=1  BreakpointsForDimension1=SPHETModel.cont_gen_mtr_trq_spdbpt  Table=SPHETModel.cont_gen_mtr_pwr_map  ExtrapMethod=Clip  UseLastTableValue=on  InternalRulePriority=Speed  RndMeth=Simplest  InputSameDT=on
  Generator Continuous Torque : Lookup_n-D  NumberOfTableDimensions=1  BreakpointsForDimension1=SPHETModel.cont_gen_mtr_trq_spdbpt  Table=SPHETModel.cont_gen_mtr_trq_map  ExtrapMethod=Clip  UseLastTableValue=on  InternalRulePriority=Speed  RndMeth=Simplest  InputSameDT=on
  Generator Efficiency : Lookup_n-D  BreakpointsForDimension1=SPHETModel.gen_mtr_trqbpt  BreakpointsForDimension2=SPHETModel.gen_mtr_spdbpt  Table=SPHETModel.gen_mtr_eff_map  ExtrapMethod=Clip  UseLastTableValue=on  InternalRulePriority=Speed  RndMeth=Simplest  InputSameDT=on
  kW2W : Gain  Gain=1000
  P_GenMtrContLim : Outport
  wires:
  gen_spd_rpm/1 -> Generator Continuous Torque/1, Generator Efficiency/2
  kW2W/1 -> Divide/1
  Generator Continuous Power kW/1 -> kW2W/1
  Generator Efficiency/1 -> Divide/2
  Generator Continuous Torque/1 -> Generator Efficiency/1
  Divide/1 -> Gain/1  "P_GenMtrContLim"
  Gain/1 -> P_GenMtrContLim/1
  Constant/1 -> Generator Continuous Power kW/1

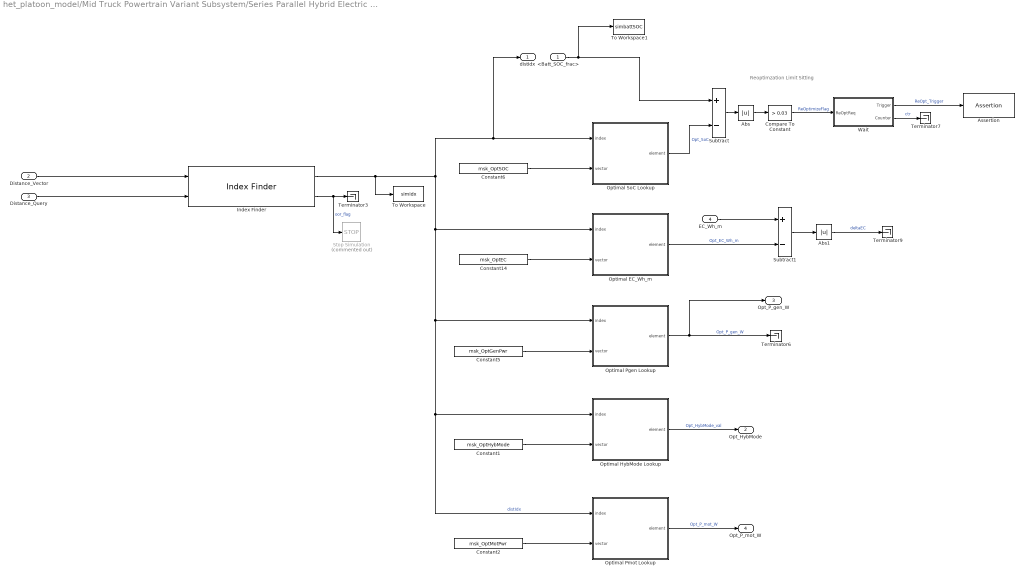
== system het_platoon_model/Mid Truck Powertrain Variant Subsystem/Series Parallel Hybrid Electric Truck/Series Parallel Hybrid Electric Truck Energy Management System/Proposed ReOpt DP Algorithm ==
  note: Reoptimzation Limit Sitting
  <Batt_SOC_frac> : Inport
  Distance_Vector : Inport  Port=2
  Distance_Query : Inport  Port=3
  EC_Wh_m : Inport  Port=4
  Abs : Abs
  Abs1 : Abs
  Assertion : Assertion  AssertionFailFcn=set_param(bdroot,'SimulationCommand','pause');  StopWhenAssertionFail=off
  Compare To Constant : simulink/Logic and Bit Operations/Compare To Constant  relop=>  const=0.03  OutDataTypeStr=boolean
  Constant1 : Constant  Value=msk_OptHybMode
  Constant14 : Constant  Value=msk_OptEC
  Constant2 : Constant  Value=msk_OptMotPwr
  Constant5 : Constant  Value=msk_OptGenPwr
  Constant6 : Constant  Value=msk_OptSOC
  Index Finder : custom_func/Index Finder  SystemSampleTime=-1
  Optimal EC_Wh_m : MATLAB Function  TreatAsAtomicUnit=on
  Optimal HybMode Lookup : MATLAB Function  TreatAsAtomicUnit=on
  Optimal Pgen Lookup : MATLAB Function  TreatAsAtomicUnit=on
  Optimal Pmot Lookup : MATLAB Function  TreatAsAtomicUnit=on
  Optimal SoC Lookup : MATLAB Function  TreatAsAtomicUnit=on
  Stop Simulation : Stop  Commented=on
  Subtract : Sum  Inputs=+-
  Subtract1 : Sum  Inputs=+-
  Terminator{3,6..7,9} (4 alike) : Terminator
  To Workspace : ToWorkspace  VariableName=simidx  SaveFormat=Timeseries  SampleTime=1
      settings: Save2DSignal=2-D array (concatenate along first dimension)
  To Workspace1 : ToWorkspace  VariableName=simbattSOC  SaveFormat=Timeseries  SampleTime=1
      settings: Save2DSignal=2-D array (concatenate along first dimension)
  Wait : Stateflow chart  TreatAsAtomicUnit=on
  distIdx : Outport
  Opt_HybMode : Outport  Port=2
  Opt_P_gen_W : Outport  Port=3
  Opt_P_mot_W : Outport  Port=4
  wires:
  Distance_Query/1 -> Index Finder/2
  <Batt_SOC_frac>/1 -> To Workspace1/1, Subtract/1
  Abs1/1 -> Terminator9/1  "deltaEC"
  Distance_Vector/1 -> Index Finder/1
  Subtract/1 -> Abs/1
  Constant6/1 -> Optimal SoC Lookup/2(vector)
  Compare To Constant/1 -> Wait/1(ReOptReq)  "ReOptimizeFlag"
  Abs/1 -> Compare To Constant/1
  Index Finder/1 -> To Workspace/1, distIdx/1, Optimal SoC Lookup/1(index), Optimal EC_Wh_m/1(index), Optimal HybMode Lookup/1(index), Optimal Pmot Lookup/1(index), Optimal Pgen Lookup/1(index)  "distIdx"
  EC_Wh_m/1 -> Subtract1/1
  Optimal SoC Lookup/1(element) -> Subtract/2  "Opt_SoC"
  Optimal EC_Wh_m/1(element) -> Subtract1/2  "Opt_EC_Wh_m"
  Subtract1/1 -> Abs1/1
  Wait/2(Counter) -> Terminator7/1  "ctr"
  Optimal Pgen Lookup/1(element) -> Opt_P_gen_W/1, Terminator6/1  "Opt_P_gen_W"
  Index Finder/2 -> Terminator3/1, Stop Simulation/1  "oor_flag"
  Constant5/1 -> Optimal Pgen Lookup/2(vector)
  Wait/1(Trigger) -> Assertion/1  "ReOpt_Trigger"
  Constant14/1 -> Optimal EC_Wh_m/2(vector)
  Constant1/1 -> Optimal HybMode Lookup/2(vector)
  Constant2/1 -> Optimal Pmot Lookup/2(vector)
  Optimal Pmot Lookup/1(element) -> Opt_P_mot_W/1  "Opt_P_mot_W"
  Optimal HybMode Lookup/1(element) -> Opt_HybMode/1  "Opt_HybMode_val"

== system het_platoon_model/Mid Truck Powertrain Variant Subsystem/Series Parallel Hybrid Electric Truck/Series Parallel Hybrid Electric Truck Energy Management System/SPHET Optimal Gear Shift Algorithm ==
  P_dem_W : Inport
  veh_spd_mps : Inport  Port=2
  Bus Creator : BusCreator  Inputs=10
  Constant : Constant  Value=eps
  Divide : Product  Inputs=*/
  Fuel LUT @ Gear 1 : Lookup_n-D  BreakpointsForDimension1=CTModel.eng_map_trq_bpt(10:end) * (CTModel.gear_ratios(1) * CTModel.fd_ratio)  BreakpointsForDimension2=(CTModel.eng_map_spd_bpt * 0.1047 * CTModel.ld_tire_rad_m)/(CTModel.gear_ratios(1) * CTModel.fd_ratio)  Table=CTModel.eng_fuel_map(10:end,:)  ExtrapMethod=Clip  UseLastTableValue=on  InternalRulePriority=Speed  RndMeth=Simplest  InputSameDT=on
  Fuel LUT @ Gear 10 : Lookup_n-D  BreakpointsForDimension1=CTModel.eng_map_trq_bpt(10:end) * (CTModel.gear_ratios(10) * CTModel.fd_ratio)  BreakpointsForDimension2=(CTModel.eng_map_spd_bpt * 0.1047 * CTModel.ld_tire_rad_m)/(CTModel.gear_ratios(10) * CTModel.fd_ratio)  Table=CTModel.eng_fuel_map(10:end,:)  ExtrapMethod=Clip  UseLastTableValue=on  InternalRulePriority=Speed  RndMeth=Simplest  InputSameDT=on
  Fuel LUT @ Gear 2 : Lookup_n-D  BreakpointsForDimension1=CTModel.eng_map_trq_bpt(10:end) * (CTModel.gear_ratios(2) * CTModel.fd_ratio)  BreakpointsForDimension2=(CTModel.eng_map_spd_bpt * 0.1047 * CTModel.ld_tire_rad_m)/(CTModel.gear_ratios(2) * CTModel.fd_ratio)  Table=CTModel.eng_fuel_map(10:end,:)  ExtrapMethod=Clip  UseLastTableValue=on  InternalRulePriority=Speed  RndMeth=Simplest  InputSameDT=on
  Fuel LUT @ Gear 3 : Lookup_n-D  BreakpointsForDimension1=CTModel.eng_map_trq_bpt(10:end) * (CTModel.gear_ratios(3) * CTModel.fd_ratio)  BreakpointsForDimension2=(CTModel.eng_map_spd_bpt * 0.1047 * CTModel.ld_tire_rad_m)/(CTModel.gear_ratios(3) * CTModel.fd_ratio)  Table=CTModel.eng_fuel_map(10:end,:)  ExtrapMethod=Clip  UseLastTableValue=on  InternalRulePriority=Speed  RndMeth=Simplest  InputSameDT=on
  Fuel LUT @ Gear 4 : Lookup_n-D  BreakpointsForDimension1=CTModel.eng_map_trq_bpt(10:end) * (CTModel.gear_ratios(4) * CTModel.fd_ratio)  BreakpointsForDimension2=(CTModel.eng_map_spd_bpt * 0.1047 * CTModel.ld_tire_rad_m)/(CTModel.gear_ratios(4) * CTModel.fd_ratio)  Table=CTModel.eng_fuel_map(10:end,:)  ExtrapMethod=Clip  UseLastTableValue=on  InternalRulePriority=Speed  RndMeth=Simplest  InputSameDT=on
  Fuel LUT @ Gear 5 : Lookup_n-D  BreakpointsForDimension1=CTModel.eng_map_trq_bpt(10:end) * (CTModel.gear_ratios(5) * CTModel.fd_ratio)  BreakpointsForDimension2=(CTModel.eng_map_spd_bpt * 0.1047 * CTModel.ld_tire_rad_m)/(CTModel.gear_ratios(5) * CTModel.fd_ratio)  Table=CTModel.eng_fuel_map(10:end,:)  ExtrapMethod=Clip  UseLastTableValue=on  InternalRulePriority=Speed  RndMeth=Simplest  InputSameDT=on
  Fuel LUT @ Gear 6 : Lookup_n-D  BreakpointsForDimension1=CTModel.eng_map_trq_bpt(10:end) * (CTModel.gear_ratios(6) * CTModel.fd_ratio)  BreakpointsForDimension2=(CTModel.eng_map_spd_bpt * 0.1047 * CTModel.ld_tire_rad_m)/(CTModel.gear_ratios(6) * CTModel.fd_ratio)  Table=CTModel.eng_fuel_map(10:end,:)  ExtrapMethod=Clip  UseLastTableValue=on  InternalRulePriority=Speed  RndMeth=Simplest  InputSameDT=on
  Fuel LUT @ Gear 7 : Lookup_n-D  BreakpointsForDimension1=CTModel.eng_map_trq_bpt(10:end) * (CTModel.gear_ratios(7) * CTModel.fd_ratio)  BreakpointsForDimension2=(CTModel.eng_map_spd_bpt * 0.1047 * CTModel.ld_tire_rad_m)/(CTModel.gear_ratios(7) * CTModel.fd_ratio)  Table=CTModel.eng_fuel_map(10:end,:)  ExtrapMethod=Clip  UseLastTableValue=on  InternalRulePriority=Speed  RndMeth=Simplest  InputSameDT=on
  Fuel LUT @ Gear 8 : Lookup_n-D  BreakpointsForDimension1=CTModel.eng_map_trq_bpt(10:end) * (CTModel.gear_ratios(8) * CTModel.fd_ratio)  BreakpointsForDimension2=(CTModel.eng_map_spd_bpt * 0.1047 * CTModel.ld_tire_rad_m)/(CTModel.gear_ratios(8) * CTModel.fd_ratio)  Table=CTModel.eng_fuel_map(10:end,:)  ExtrapMethod=Clip  UseLastTableValue=on  InternalRulePriority=Speed  RndMeth=Simplest  InputSameDT=on
  Fuel LUT @ Gear 9 : Lookup_n-D  BreakpointsForDimension1=CTModel.eng_map_trq_bpt(10:end) * (CTModel.gear_ratios(9) * CTModel.fd_ratio)  BreakpointsForDimension2=(CTModel.eng_map_spd_bpt * 0.1047 * CTModel.ld_tire_rad_m)/(CTModel.gear_ratios(9) * CTModel.fd_ratio)  Table=CTModel.eng_fuel_map(10:end,:)  ExtrapMethod=Clip  UseLastTableValue=on  InternalRulePriority=Speed  RndMeth=Simplest  InputSameDT=on
  Loaded Tire Radius m : Gain  Gain=msk_tire_radius_m
  Minimum Function : MATLAB Function  TreatAsAtomicUnit=on
  Switch : Switch  Criteria=u2 > Threshold
  Transmission Efficiency : Gain  Gain=1/msk_trns_eff_avg
  init_gear : Constant  Value=msk_init_gear
  opt_gear : Outport
  wires:
  Transmission Efficiency/1 -> Divide/1
  P_dem_W/1 -> Loaded Tire Radius m/1
  Fuel LUT @ Gear 5/1 -> Bus Creator/5  "m_fuel_Gear_5"
  Fuel LUT @ Gear 6/1 -> Bus Creator/6  "m_fuel_Gear_6"
  Bus Creator/1 -> Minimum Function/1(m_fuel_vec)
  Fuel LUT @ Gear 2/1 -> Bus Creator/2  "m_fuel_Gear_2"
  Fuel LUT @ Gear 8/1 -> Bus Creator/8  "m_fuel_Gear_8"
  Fuel LUT @ Gear 9/1 -> Bus Creator/9  "m_fuel_Gear_9"
  Divide/1 -> Fuel LUT @ Gear 1/1, Fuel LUT @ Gear 2/1, Fuel LUT @ Gear 3/1, Fuel LUT @ Gear 4/1, Fuel LUT @ Gear 5/1, Fuel LUT @ Gear 6/1, Fuel LUT @ Gear 7/1, Fuel LUT @ Gear 8/1, Fuel LUT @ Gear 9/1, Fuel LUT @ Gear 10/1
  Fuel LUT @ Gear 3/1 -> Bus Creator/3  "m_fuel_Gear_3"
  Switch/1 -> Divide/2
  Fuel LUT @ Gear 10/1 -> Bus Creator/10  "m_fuel_Gear_10"
  Minimum Function/1(opt_gear) -> opt_gear/1
  Fuel LUT @ Gear 7/1 -> Bus Creator/7  "m_fuel_Gear_7"
  Fuel LUT @ Gear 1/1 -> Bus Creator/1  "m_fuel_Gear_1"
  Constant/1 -> Switch/3
  veh_spd_mps/1 -> Fuel LUT @ Gear 2/2, Fuel LUT @ Gear 3/2, Fuel LUT @ Gear 4/2, Fuel LUT @ Gear 5/2, Fuel LUT @ Gear 6/2, Fuel LUT @ Gear 7/2, Fuel LUT @ Gear 8/2, Fuel LUT @ Gear 9/2, Fuel LUT @ Gear 10/2, Fuel LUT @ Gear 1/2, Switch/1, Switch/2
  init_gear/1 -> Minimum Function/2(prev_gear)
  Loaded Tire Radius m/1 -> Transmission Efficiency/1
  Fuel LUT @ Gear 4/1 -> Bus Creator/4  "m_fuel_Gear_4"

== system het_platoon_model/Mid Truck Powertrain Variant Subsystem/Series Parallel Hybrid Electric Truck/Series Parallel Hybrid Electric Powertrain Power Loss Model/A123 ESS Model/OCV_Battery ==
  note: Intial SOC value goes in this memory block
  Current : Inport
  Add : Sum
  Constant : Constant  Value=msk_batt_Ns
  Constant1 : Constant  Value=msk_cell_Q_Ah * msk_batt_Np
  Constant2 : Constant  Value=msk_batt_Nmod
  Divide : Product  Inputs=*/
  Gain : Gain  Gain=msk_t_step/3600
  Memory : Memory  InitialCondition=msk_batt_soc_init  InheritSampleTime=on  LinearizeAsDelay=on
  OCV Function : MATLAB Function  TreatAsAtomicUnit=on
  Product : Product  Inputs=3
  SOC_calc : Outport
  Current_pt : Outport  Port=2
  BattVolt_calc : Outport  Port=3
  wires:
  Product/1 -> BattVolt_calc/1  "BattVolt_calc"
  Divide/1 -> Add/2
  Constant/1 -> Product/2
  Add/1 -> OCV Function/1(soc), Memory/1, SOC_calc/1  "SOC_calc"
  Constant1/1 -> Divide/2
  OCV Function/1(ocv) -> Product/1  "OCV_calc"
  Constant2/1 -> Product/3
  Memory/1 -> Add/1
  Gain/1 -> Divide/1
  Current/1 -> Gain/1, Current_pt/1, OCV Function/2(current)

== system het_platoon_model/Mid Truck Powertrain Variant Subsystem/Series Parallel Hybrid Electric Truck/Series Parallel Hybrid Electric Powertrain Power Loss Model/A123 ESS Model/R0 Resistance ==
  SOC : Inport
  Current : Inport  Port=2
  Compare To Zero : simulink/Logic and Bit Operations/Compare To Zero  relop=>  OutDataTypeStr=boolean
  Product : Product
  R0 LUT Chg : Lookup_n-D  NumberOfTableDimensions=1  BreakpointsForDimension1=msk_batt_soc_bpt  Table=msk_batt_R0 * 0.05  ExtrapMethod=Clip  UseLastTableValue=on  InternalRulePriority=Speed  RndMeth=Simplest  InputSameDT=on
  R0 LUT Dchg : Lookup_n-D  NumberOfTableDimensions=1  BreakpointsForDimension1=msk_batt_soc_bpt  Table=msk_batt_R0 * 0.25  ExtrapMethod=Clip  UseLastTableValue=on  InternalRulePriority=Speed  RndMeth=Simplest  InputSameDT=on
  Switch : Switch  Criteria=u2 > Threshold
  V_R0 : Outport
  wires:
  R0 LUT Dchg/1 -> Switch/3  "R0"
  Compare To Zero/1 -> Switch/2
  Switch/1 -> Product/1
  Product/1 -> V_R0/1
  Current/1 -> Product/2, Compare To Zero/1
  SOC/1 -> R0 LUT Dchg/1, R0 LUT Chg/1
  R0 LUT Chg/1 -> Switch/1  "R0"

== system het_platoon_model/Mid Truck Powertrain Variant Subsystem/Series Parallel Hybrid Electric Truck/Series Parallel Hybrid Electric Powertrain Power Loss Model/A123 ESS Model/R1_C1 Circuit ==
  SOC : Inport
  Current : Inport  Port=2
  Add1 : Sum
  C1 LUT : Lookup_n-D  NumberOfTableDimensions=1  BreakpointsForDimension1=msk_batt_soc_bpt  Table=msk_batt_C1  ExtrapMethod=Clip  UseLastTableValue=on  InternalRulePriority=Speed  RndMeth=Simplest  InputSameDT=on
  Discrete-Time Integrator : DiscreteIntegrator  SampleTime=-1  ICPrevOutput=DiscIntNeverNeededParam  ICPrevScaledInput=DiscIntNeverNeededParam
  Divide : Product  Inputs=*/
  Divide1 : Product  Inputs=*/
  Product : Product
  R1 LUT : Lookup_n-D  NumberOfTableDimensions=1  BreakpointsForDimension1=msk_batt_soc_bpt  Table=msk_batt_R1  ExtrapMethod=Clip  UseLastTableValue=on  InternalRulePriority=Speed  RndMeth=Simplest  InputSameDT=on
  U_PC : Outport
  wires:
  Current/1 -> Divide/1
  Add1/1 -> Discrete-Time Integrator/1  "U_PC_derivative"
  Discrete-Time Integrator/1 -> Divide1/1, U_PC/1  "U_PC"
  R1 LUT/1 -> Product/1
  Divide/1 -> Add1/2
  C1 LUT/1 -> Divide/2, Product/2
  Divide1/1 -> Add1/1
  SOC/1 -> C1 LUT/1, R1 LUT/1
  Product/1 -> Divide1/2

== system het_platoon_model/Mid Truck Powertrain Variant Subsystem/Series Parallel Hybrid Electric Truck/Series Parallel Hybrid Electric Powertrain Power Loss Model/A123 ESS Model/R2_C2 Circuit ==
  SOC : Inport
  Current : Inport  Port=2
  Add1 : Sum
  C2 LUT : Lookup_n-D  NumberOfTableDimensions=1  BreakpointsForDimension1=msk_batt_soc_bpt  Table=msk_batt_C2  ExtrapMethod=Clip  UseLastTableValue=on  InternalRulePriority=Speed  RndMeth=Simplest  InputSameDT=on
  Discrete-Time Integrator : DiscreteIntegrator  SampleTime=-1  ICPrevOutput=DiscIntNeverNeededParam  ICPrevScaledInput=DiscIntNeverNeededParam
  Divide : Product  Inputs=*/
  Divide1 : Product  Inputs=*/
  Product : Product
  R2 LUT : Lookup_n-D  NumberOfTableDimensions=1  BreakpointsForDimension1=msk_batt_soc_bpt  Table=msk_batt_R2  ExtrapMethod=Clip  UseLastTableValue=on  InternalRulePriority=Speed  RndMeth=Simplest  InputSameDT=on
  U_PA : Outport
  wires:
  Current/1 -> Divide/1
  Add1/1 -> Discrete-Time Integrator/1  "U_PA_derivative"
  Discrete-Time Integrator/1 -> Divide1/1, U_PA/1  "U_PA"
  R2 LUT/1 -> Product/1
  Divide/1 -> Add1/2
  C2 LUT/1 -> Divide/2, Product/2
  Divide1/1 -> Add1/1
  SOC/1 -> C2 LUT/1, R2 LUT/1
  Product/1 -> Divide1/2
